simulink model "laba11"  (R2023a)
settings: Solver=VariableStepAuto  StartTime=0.0  StopTime=10  RelTol=1e-3
values from neighbouring files (symbols this model uses):
  m = m + 1    (= 2)    [TMO5liubimov.m]    (also in laba2.m = 14; laba3.m = 200; test.m = 5)
  n = 31    [laba2.m]    (also in test.m = 7)
settings Model: Creator=Evangelina  LastModifiedBy=PC
settings RTWCC: GPUComputeCapability=5.0

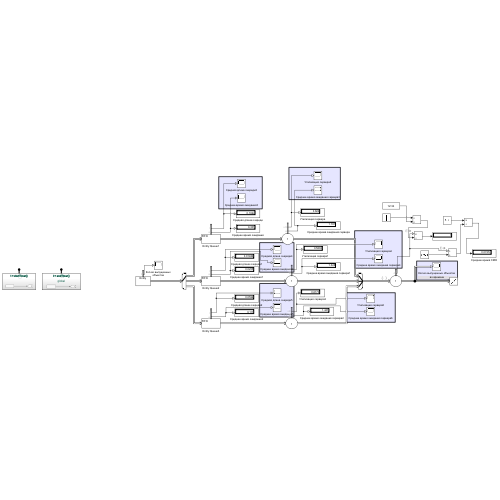
[thumbnail: Simulink's stored preview of the top-level diagram]
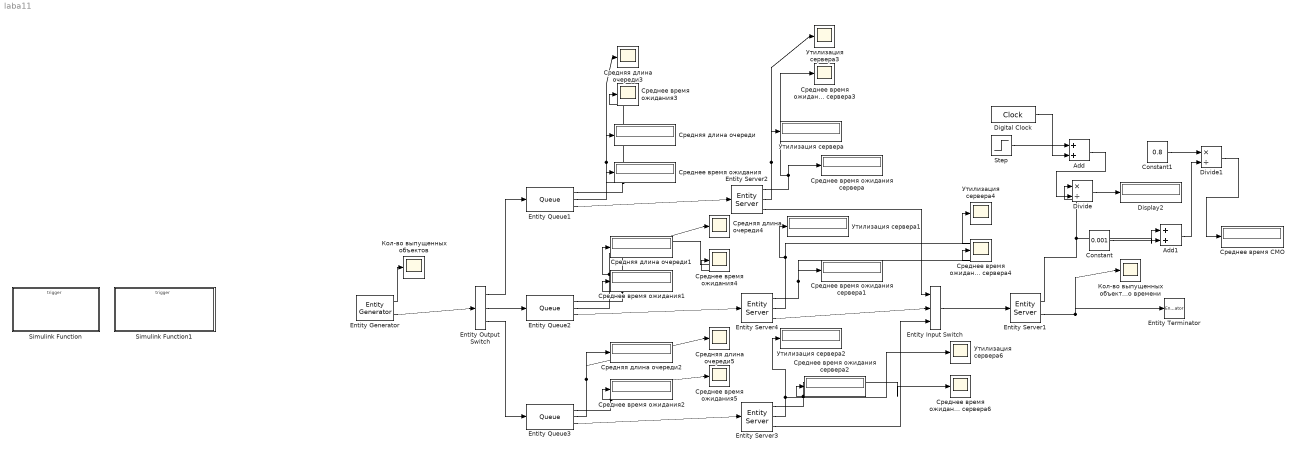
== system laba11 ==
  Add : Sum
  Add1 : Sum
  Constant : Constant  Value=0.001
  Constant1 : Constant  Value=0.8
  Digital Clock : DigitalClock
  Display2 : Display
  Divide : Product  Inputs=*/
  Divide1 : Product  Inputs=*/
  Entity Input Switch : EntityInputSwitch  InputPortMessageModes=m,m,m  OutputPortMessageModes=m  NumberInputPorts=3
      settings: InputPortMap=u1,u2,u3
  Entity Output Switch : EntityOutputSwitch  InputPortMessageModes=m  OutputPortMessageModes=m,m,m  NumberOutputPorts=3  SwitchingCriterion=Round robin  SwitchAttributeName=Attribute1
      settings: OutputPortMap=o0,o1,o2
  Entity Generator : EntityGenerator  OutputPortMessageModes=n,m  TimeSource=MATLAB action  IntergenerationTimeAction=|  AttributeName=SMOTime  AttributeInitialValue=0  NumberEntitiesDeparted=on  EntityType=Structured  EntityTypeName=Entity
      | persistent rngInit;
      | if isempty(rngInit)
      |     rng(12345);      
      |     rngInit = true;
      | end
      | 
      | mean = 1; 
      | lambda = 1 / mean;  
      | dt = -log(rand()) / lambda;
      settings: OutputPortMap=o0,o3
  Entity Queue1 : Queue  InputPortMessageModes=m  OutputPortMessageModes=n,n,m  AverageWait=on  AverageQueueLength=on
      settings: OutputPortMap=o2,o3,o5
  Entity Queue2 : Queue  InputPortMessageModes=m  OutputPortMessageModes=n,n,m  AverageWait=on  AverageQueueLength=on
      settings: OutputPortMap=o2,o3,o5
  Entity Queue3 : Queue  InputPortMessageModes=m  OutputPortMessageModes=n,n,m  AverageWait=on  AverageQueueLength=on
      settings: OutputPortMap=o2,o3,o5
  Entity Server1 : EntityServer  InputPortMessageModes=m  OutputPortMessageModes=n,m  Capacity=1  ServiceTimeSource=MATLAB action  EntryAction=entity.SMOTime = startTimer();  NumberEntitiesDeparted=on
      settings: OutputPortMap=o0,o9
  Entity Server2 : EntityServer  InputPortMessageModes=m  OutputPortMessageModes=n,n,m  Capacity=1  AverageWait=on  Utilization=on
      settings: OutputPortMap=o4,o5,o9
  Entity Server3 : EntityServer  InputPortMessageModes=m  OutputPortMessageModes=n,n,m  Capacity=1  AverageWait=on  Utilization=on
      settings: OutputPortMap=o4,o5,o9
  Entity Server4 : EntityServer  InputPortMessageModes=m  OutputPortMessageModes=n,n,m  Capacity=1  AverageWait=on  Utilization=on
      settings: OutputPortMap=o4,o5,o9
  Entity Terminator : EntityTerminator  InputPortMessageModes=m
  Simulink Function : Subsystem  TreatAsAtomicUnit=on
  Simulink Function1 : Subsystem  TreatAsAtomicUnit=on
  Step : Step  SampleTime=0
  Кол-во выпущенных объектов : Scope
  Кол-во выпущенных объектов во времени : Scope
  Среднее время СМО : Display
  Среднее время ожидания : Display
  Среднее время ожидания сервера : Display
  Среднее время ожидания сервера1 : Display
  Среднее время ожидания сервера2 : Display
  Среднее время ожидания сервера3 : Scope
  Среднее время ожидания сервера4 : Scope
  Среднее время ожидания сервера6 : Scope
  Среднее время ожидания1 : Display
  Среднее время ожидания2 : Display
  Среднее время ожидания3 : Scope
  Среднее время ожидания4 : Scope
  Среднее время ожидания5 : Scope
  Средняя длина очереди : Display
  Средняя длина очереди1 : Display
  Средняя длина очереди2 : Display
  Средняя длина очереди3 : Scope
  Средняя длина очереди4 : Scope
  Средняя длина очереди5 : Scope
  Утилизация сервера : Display
  Утилизация сервера1 : Display
  Утилизация сервера2 : Display
  Утилизация сервера3 : Scope
  Утилизация сервера4 : Scope
  Утилизация сервера6 : Scope
  wires:
  Constant1/1 -> Divide1/1
  Step/1 -> Add/1
  Divide/1 -> Display2/1
  Add/1 -> Divide/2
  Divide1/1 -> Среднее время СМО/1
  Entity Server1/1 -> Add1/1, Divide/1
  Constant/1 -> Add1/2
  Digital Clock/1 -> Add/2
  Add1/1 -> Divide1/2
  Entity Server1/2 -> Entity Terminator/1, Кол-во выпущенных объектов во времени/1
  Entity Generator/1 -> Кол-во выпущенных объектов/1
  Entity Generator/2 -> Entity Output Switch/1
  Entity Queue1/2 -> Средняя длина очереди3/1, Средняя длина очереди/1
  Entity Queue1/1 -> Среднее время ожидания3/1, Среднее время ожидания/1
  Entity Server2/1 -> Среднее время ожидания сервера3/1, Среднее время ожидания сервера/1
  Entity Server2/2 -> Утилизация сервера3/1, Утилизация сервера/1
  Entity Output Switch/1 -> Entity Queue1/1
  Entity Queue1/3 -> Entity Server2/1
  Entity Server2/3 -> Entity Input Switch/1
  Entity Input Switch/1 -> Entity Server1/1
  Entity Queue2/1 -> Среднее время ожидания4/1, Среднее время ожидания1/1
  Entity Queue2/2 -> Средняя длина очереди4/1, Средняя длина очереди1/1
  Entity Server4/2 -> Утилизация сервера4/1, Утилизация сервера1/1
  Entity Server4/1 -> Среднее время ожидания сервера4/1, Среднее время ожидания сервера1/1
  Entity Server4/3 -> Entity Input Switch/2
  Entity Queue2/3 -> Entity Server4/1
  Entity Output Switch/2 -> Entity Queue2/1
  Entity Server3/2 -> Утилизация сервера6/1, Утилизация сервера2/1
  Entity Queue3/3 -> Entity Server3/1
  Entity Queue3/2 -> Средняя длина очереди5/1, Средняя длина очереди2/1
  Entity Queue3/1 -> Среднее время ожидания5/1, Среднее время ожидания2/1
  Entity Server3/1 -> Среднее время ожидания сервера6/1, Среднее время ожидания сервера2/1
  Entity Output Switch/3 -> Entity Queue3/1
  Entity Server3/3 -> Entity Input Switch/3

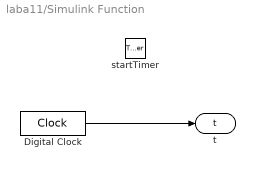
== system laba11/Simulink Function ==
  startTimer : TriggerPort  TriggerType=function-call  IsSimulinkFunction=on  FunctionName=startTimer  FunctionVisibility=scoped  VariantControl=(inherit)
  Digital Clock : DigitalClock  SampleTime=-1
  t : ArgOut  DisableCoverage=on  ArgumentName=t
  wires:
  Digital Clock/1 -> t/1

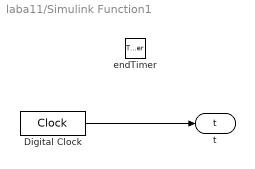
== system laba11/Simulink Function1 ==
  endTimer : TriggerPort  TriggerType=function-call  IsSimulinkFunction=on  FunctionName=endTimer  VariantControl=(inherit)
  Digital Clock : DigitalClock  SampleTime=-1
  t : ArgOut  DisableCoverage=on  ArgumentName=t
  wires:
  Digital Clock/1 -> t/1
